simulink library "IsourcePower_lib"  (Simulink 8.1)
settings: Solver=ode45  SolverMode=SingleTasking  StartTime=0.0  StopTime=10.0  RelTol=1e-3
values from neighbouring files (symbols this model uses):
  Igrid = Pgrid/Vgrid/3    [Software_BESS_init.m]
  Ls_ess = Ls_ess_PU*Ls_ess_base    (= 0.000249351232441)    [Software_BESS_init.m]
  PUIMax = 1.2    [Software_BESS_init.m]
  Rs_ess = Rs_ess_PU*Rs_ess_base    (= 0.00497664)    [Software_BESS_init.m]
  sampdT = Tc    (= 0.0001)    [Software_BESS_init.m]
  Tc = Ts    (= 0.0001)    [Software_BESS_init.m]
  Ts = 100e-6    (= 0.0001)    [Software_BESS_init.m]
  Vgrid = 480/sqrt(3)    [Software_BESS_init.m]
undefined symbols (not defined in the file or in its folder): DiscIntNeverNeededParam, gcbh, sps, sps_rtmsupport
undefined symbols (not defined in the file): paramPLLControlD, paramPLLControlI, paramPLLControlP, PLLFreqChangeRateMax, PLLFreqCutOff
libraries: simulink x13, powerlib x12, powerlib_meascontrol x11, debounce_lib x8, powerlib_extras x7
settings Model: Creator=ch24070  LastModifiedBy=pkoralew  CovMetricSettings=dwe  CovHtmlReporting=off  covSaveCumulativeToWorkspaceVar=off  CovSaveSingleToWorkspaceVar=off  CovExternalEMLEnable=on

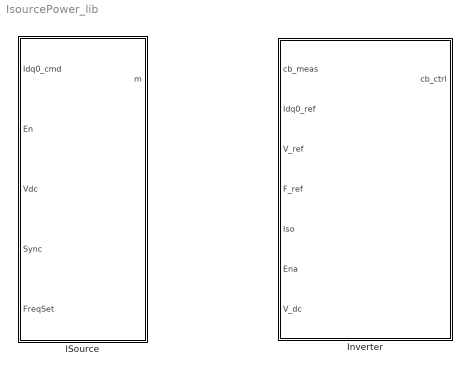
== system IsourcePower_lib ==
  ISource : Subsystem
  Inverter : Subsystem

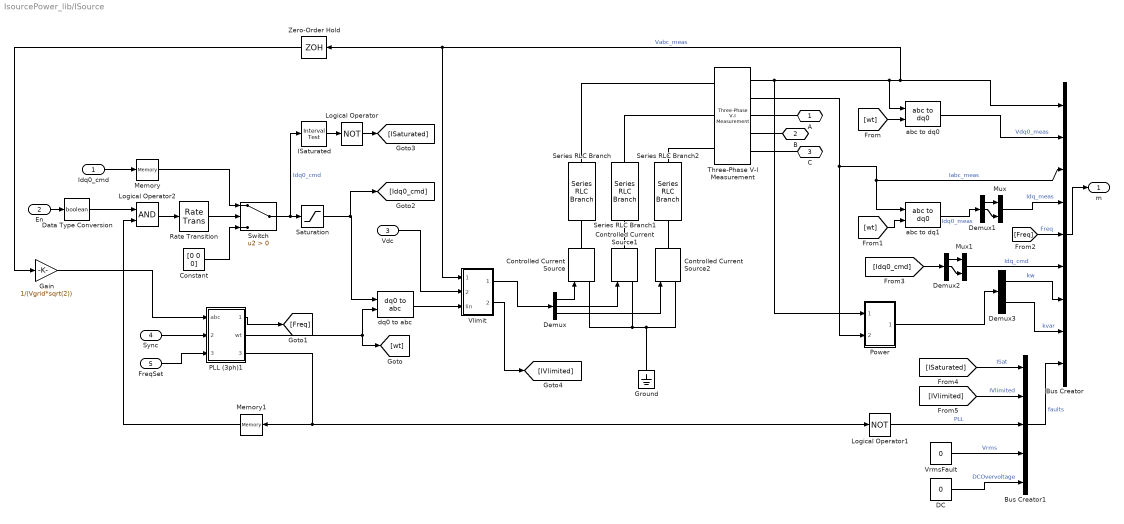
== system IsourcePower_lib/ISource ==
  Idq0_cmd : Inport
  En : Inport  Port=2
  Vdc : Inport  Port=3
  Sync : Inport  Port=4
  FreqSet : Inport  Port=5
  Bus Creator : BusCreator  Inputs=9
  Bus Creator1 : BusCreator  Inputs=5
  Constant : Constant  Value=[0 0 0]
  Controlled Current Source : powerlib/Electrical Sources/Controlled Current Source  Initialize=on  Source_Type=AC  Amplitude=0  Phase=0  Frequency=0  Measurements=None
  Controlled Current Source1 : powerlib/Electrical Sources/Controlled Current Source  Initialize=on  Source_Type=AC  Amplitude=0  Phase=0  Frequency=0  Measurements=None
  Controlled Current Source2 : powerlib/Electrical Sources/Controlled Current Source  Initialize=on  Source_Type=AC  Amplitude=0  Phase=0  Frequency=0  Measurements=None
  DC : Constant  Value=0
  Data Type Conversion : DataTypeConversion  OutDataTypeStr=boolean
  Demux : Demux  Outputs=3
  Demux1 : Demux  Outputs=3
  Demux2 : Demux  Outputs=3
  Demux3 : Demux  Outputs=2
  Gain : Gain  Gain=1/(Vgrid*sqrt(2))
  Ground : powerlib/Elements/Ground  LConnTagsString=a
  ISaturated : simulink/Logic and Bit Operations/Interval Test  IntervalClosedRight=on  uplimit=Igrid*sqrt(2)*PUIMax  IntervalClosedLeft=on  lowlimit=-Igrid*sqrt(2)*PUIMax  OutDataTypeStr=boolean
  Logical Operator : Logic  Operator=NOT  AllPortsSameDT=off  OutDataTypeStr=boolean
  Logical Operator1 : Logic  Operator=NOT  AllPortsSameDT=off  OutDataTypeStr=boolean
  Logical Operator2 : Logic  AllPortsSameDT=off  OutDataTypeStr=boolean
  Memory : Memory
  Memory1 : Memory
  Mux : Mux  Inputs=2
  Mux1 : Mux  Inputs=2
  PLL (3ph)1 : Subsystem  DialogController=POWERSYS.PowerSysDialog  LoadFcn=sps_rtmsupport('LoadFcn', gcbh);  StartFcn=sps_rtmsupport('StartFcn', gcbh);  StopFcn=sps_rtmsupport('StopFcn', gcbh);  mask(PLL (3ph)){Fmin=45, Par_Init=[0, 60], ParK=[paramPLLControlP, paramPLLControlI, paramPLLControlD], TcD=Tc, MaxRateChangeFreq=PLLFreqChangeRateMax, FilterCutOffFreq=PLLFreqCutOff, Ts=Tc, AGC=off}
      mask prompts: Fmin "Minimum frequency (Hz):"; Par_Init "Initial inputs [ Phase (degrees), Frequency (Hz) ]:"; ParK "Regulator gains [ Kp, Ki, Kd ]:"; TcD "Time constant for derivative action (s):"; MaxRateChangeFreq "Maximum rate of change of frequency (Hz/s):"; FilterCutOffFreq "Filter cut-off frequency for frequency measurement (Hz):"; Ts "Sample time:"; AGC "Enable automatic gain control"
      mask help:
      | This Phase Locked Loop (PLL) system can be used  to synchronize on a set of variable frequency, three-phase sinusoidal signals. If the Automatic Gain Control is enabled, the input (phase error) of the PLL regulator is scaled according to the input signals magnitude.
      |
      | For optimal performance, set regulator gains [ Kp Ki  Kd ] = [ 180  3200  1 ] and check the Enable Automatic Gain Control parameter.
      |
      | Input : Vector containing the normalized three-phase signals [Va Vb Vc]
      | Output 1:  Measured frequency (Hz) = w/(2pi)
      | Output 2:  Ramp w.t varying between  0 and 2*pi, synchronized on zero crossings of the fundamental (positive-sequence) of phase A.
      mask init:
      | %block=gcb;
      | %[WantBlockChoice,Ts,sps] = powericon('PLL3phInit',block,Fmin,Par_Init,ParK,TcD, MaxRateChangeFreq, FilterCutOffFreq, AGC,Ts);
      | %powericon('SetInternalModels','set',block,WantBlockChoice);
      settings: CopyFcn=sps_rtmsupport('CopyFcn', gcbh);  DeleteFcn=sps_rtmsupport('DeleteFcn', gcbh);  UndoDeleteFcn=sps_rtmsupport('UndoDeleteFcn', gcbh);  ModelCloseFcn=sps_rtmsupport('ModelCloseFcn', gcbh);  PreSaveFcn=sps_rtmsupport('PreSaveFcn', gcbh);  PostSaveFcn=sps_rtmsupport('PostSaveFcn', gcbh);  NameChangeFcn=sps_rtmsupport('NameChangeFcn', gcbh);  PreCopyFcn=sps_rtmsupport('PreCopyFcn', gcbh);  CloseFcn=sps_rtmsupport('CloseFcn', gcbh);  PreDeleteFcn=sps_rtmsupport('PreDeleteFcn', gcbh);
      settings: OpenFcn=|
      | power_openblockproxy();
      | sps_rtmsupport('OpenFcn', gcbh, [8]);
      mask Help: helpview(psbhelp);
  Power : Subsystem
  Rate Transition : RateTransition  OutPortSampleTime=Tc
  Saturation : Saturate  UpperLimit=Igrid*sqrt(2)*PUIMax  LowerLimit=-Igrid*sqrt(2)*PUIMax
  Series RLC Branch : powerlib/Elements/Series RLC Branch  LConnTagsString=__new0  RConnTagsString=__new0  BranchType=R  Resistance=1e-3  Inductance=0  SetiL0=off  InitialCurrent=0  Capacitance=0  Setx0=off  InitialVoltage=0  Measurements=None
  Series RLC Branch1 : powerlib/Elements/Series RLC Branch  LConnTagsString=__new0  RConnTagsString=__new0  BranchType=R  Resistance=1e-3  Inductance=0  SetiL0=off  InitialCurrent=0  Capacitance=0  Setx0=off  InitialVoltage=0  Measurements=None
  Series RLC Branch2 : powerlib/Elements/Series RLC Branch  LConnTagsString=__new0  RConnTagsString=__new0  BranchType=R  Resistance=1e-3  Inductance=0  SetiL0=off  InitialCurrent=0  Capacitance=0  Setx0=off  InitialVoltage=0  Measurements=None
  Switch : Switch  Criteria=u2 > Threshold
  Three-Phase V-I Measurement : powerlib/Measurements/Three-Phase V-I Measurement  VoltageMeasurement=phase-to-ground  SetLabelV=off  LabelV=Vabc  Vpu=off  VpuLL=off  CurrentMeasurement=yes  SetLabelI=off  LabelI=Iabc  Ipu=off  Pbase=100e6  Vbase=500e3  OutputType=Complex  PhasorSimulation=off  PSBequivalent=0
  Vlimit : Subsystem
  VrmsFault : Constant  Value=0
  Zero-Order Hold : ZeroOrderHold  SampleTime=Tc
  abc to dq0 : powerlib_meascontrol/Transformations/abc to dq0  Alignment=90 degrees behind phase A axis
  abc to dq1 : powerlib_meascontrol/Transformations/abc to dq0  Alignment=90 degrees behind phase A axis
  dq0 to abc : powerlib_meascontrol/Transformations/dq0 to abc  Alignment=90 degrees behind phase A axis
  A : PMIOPort  Port=1  Side=Right
  B : PMIOPort  Port=2  Side=Right
  C : PMIOPort  Port=3  Side=Right
  m : Outport
  wires:
  Memory1/1 -> Logical Operator2/2
  Data Type Conversion/1 -> Logical Operator2/1
  Logical Operator2/1 -> Rate Transition/1
  PLL (3ph)1/3(Lock) -> Logical Operator1/1, Memory1/1
  FreqSet/1 -> PLL (3ph)1/3(FreqSet)
  Sync/1 -> PLL (3ph)1/2(Sync)
  Logical Operator/1 -> [ISaturated]
  DC/1 -> Bus Creator1/5  "DCOvervoltage"
  Logical Operator1/1 -> Bus Creator1/3  "PLL"
  VrmsFault/1 -> Bus Creator1/4  "Vrms"
  [IVlimited] -> Bus Creator1/2  "IVlimited"
  Vlimit/2(Sat) -> [IVlimited]
  [ISaturated] -> Bus Creator1/1  "ISat"
  ISaturated/1 -> Logical Operator/1
  [Idq0_cmd] -> Demux2/1
  Power/1(Out1) -> Demux3/1
  Bus Creator1/1 -> Bus Creator/9  "faults"
  Vlimit/1(Ilim) -> Demux/1
  dq0 to abc/1 -> Vlimit/3(Iin)
  Vdc/1 -> Vlimit/2(Vdc)
  Saturation/1 -> dq0 to abc/1, [Idq0_cmd]
  Demux3/1 -> Bus Creator/7  "kw"
  Demux3/2 -> Bus Creator/8  "kvar"
  Bus Creator/1 -> m/1
  [Freq] -> Bus Creator/5  "Freq"
  Memory/1 -> Switch/1
  PLL (3ph)1/2(wt) -> dq0 to abc/2, [wt]
  Gain/1 -> PLL (3ph)1/1(abc)
  PLL (3ph)1/1(Freq) -> [Freq]
  Zero-Order Hold/1 -> Gain/1
  Constant/1 -> Switch/3
  En/1 -> Data Type Conversion/1
  abc to dq1/1 -> Demux1/1  "Idq0_meas"
  [wt] -> abc to dq1/2
  abc to dq0/1 -> Bus Creator/2  "Vdq0_meas"
  [wt] -> abc to dq0/2
  Three-Phase V-I Measurement/2 -> abc to dq1/1, Bus Creator/3, Power/2(In2)  "Iabc_meas"
  Three-Phase V-I Measurement/1 -> Zero-Order Hold/1, Vlimit/1(Vabc), Bus Creator/1, abc to dq0/1, Power/1(In1)  "Vabc_meas"
  Switch/1 -> Saturation/1, ISaturated/1  "Idq0_cmd"
  Demux/1 -> Controlled Current Source/1
  Demux/2 -> Controlled Current Source1/1
  Demux/3 -> Controlled Current Source2/1
  Rate Transition/1 -> Switch/2
  Demux1/1 -> Mux/1
  Demux1/2 -> Mux/2
  Demux2/1 -> Mux1/1
  Demux2/2 -> Mux1/2
  Mux1/1 -> Bus Creator/6  "Idq_cmd"
  Mux/1 -> Bus Creator/4  "Idq_meas"
  Idq0_cmd/1 -> Memory/1
  connections:
  Three-Phase V-I Measurement/RConn3 -- C/RConn1
  Three-Phase V-I Measurement/RConn1 -- A/RConn1
  Three-Phase V-I Measurement/RConn2 -- B/RConn1
  Three-Phase V-I Measurement/LConn1 -- Series RLC Branch/LConn1
  Three-Phase V-I Measurement/LConn3 -- Series RLC Branch2/LConn1
  Three-Phase V-I Measurement/LConn2 -- Series RLC Branch1/LConn1
  Controlled Current Source/RConn1 -- Series RLC Branch/RConn1
  Controlled Current Source1/RConn1 -- Series RLC Branch1/RConn1
  Controlled Current Source2/RConn1 -- Series RLC Branch2/RConn1
  Controlled Current Source/LConn1 -- Controlled Current Source1/LConn1 -- Controlled Current Source2/LConn1 -- Ground/LConn1

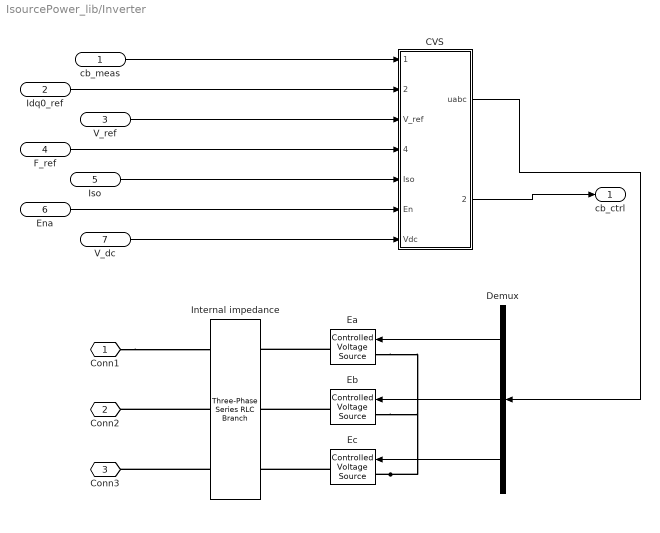
== system IsourcePower_lib/Inverter ==
  cb_meas : Inport
  Idq0_ref : Inport  Port=2
  V_ref : Inport  Port=3
  F_ref : Inport  Port=4
  Iso : Inport  Port=5
  Ena : Inport  Port=6
  V_dc : Inport  Port=7
  CVS : Subsystem
  Demux : Demux  Outputs=3
  Ea : powerlib/Electrical Sources/Controlled Voltage Source  Initialize=on  Source_Type=DC  Amplitude=0  Phase=0  Frequency=0  Measurements=None
  Eb : powerlib/Electrical Sources/Controlled Voltage Source  Initialize=on  Source_Type=DC  Amplitude=0  Phase=0  Frequency=0  Measurements=None
  Ec : powerlib/Electrical Sources/Controlled Voltage Source  Initialize=on  Source_Type=DC  Amplitude=0  Phase=0  Frequency=0  Measurements=None
  Internal impedance : powerlib/Elements/Three-Phase Series RLC Branch  LConnTagsString=A|B|C  RConnTagsString=A|B|C  BranchType=RL  Resistance=Rs_ess  Inductance=Ls_ess  Capacitance=1e-6  Measurements=None
  Conn1 : PMIOPort  Port=1  Side=Right
  Conn2 : PMIOPort  Port=2  Side=Right
  Conn3 : PMIOPort  Port=3  Side=Right
  cb_ctrl : Outport
  wires:
  V_ref/1 -> CVS/3(V_ref)
  cb_meas/1 -> CVS/1(cb_meas)
  CVS/2(cb_control) -> cb_ctrl/1
  Iso/1 -> CVS/5(Iso)
  V_dc/1 -> CVS/7(Vdc)
  F_ref/1 -> CVS/4(FreqSet)
  Ena/1 -> CVS/6(En)
  CVS/1(uabc) -> Demux/1
  Demux/1 -> Ea/1
  Demux/2 -> Eb/1
  Demux/3 -> Ec/1
  Idq0_ref/1 -> CVS/2(idq0_ref)
  connections:
  Ec/LConn1 -- Eb/LConn1 -- Ea/LConn1
  Ec/RConn1 -- Internal impedance/LConn3
  Eb/RConn1 -- Internal impedance/LConn2
  Ea/RConn1 -- Internal impedance/LConn1
  Conn1/RConn1 -- Internal impedance/RConn1
  Internal impedance/RConn2 -- Conn2/RConn1
  Internal impedance/RConn3 -- Conn3/RConn1

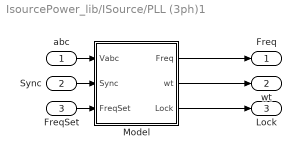
== system IsourcePower_lib/ISource/PLL (3ph)1 ==
  abc : Inport  PortDimensions=3  SampleTime=Ts
  Sync : Inport  Port=2  SampleTime=Ts
  FreqSet : Inport  Port=3  SampleTime=Ts
  Model : Subsystem  DialogController=POWERSYS.PowerSysDialog
  Freq : Outport  SampleTime=Ts
  wt : Outport  Port=2  SampleTime=Ts
  Lock : Outport  Port=3  SampleTime=Ts
  wires:
  Model/2(wt) -> wt/1
  Model/1(Freq) -> Freq/1
  FreqSet/1 -> Model/3(FreqSet)
  Sync/1 -> Model/2(Sync)
  abc/1 -> Model/1(Vabc)
  Model/3(Lock) -> Lock/1

== system IsourcePower_lib/ISource/Power ==
  In1 : Inport
  In2 : Inport  Port=2
  3-phase  Instantaneous  Active & Reactive Power : powerlib_extras/Measurements/3-phase  Instantaneous  Active & Reactive Power
  Discrete  Mean value2 : powerlib_extras/Discrete Measurements/Discrete  Mean value  Freq=60  Vinit=0  Ts=Ts
  Gain1 : Gain  Gain=(1/1000)
  Out1 : Outport
  wires:
  In1/1 -> 3-phase  Instantaneous  Active & Reactive Power/1
  In2/1 -> 3-phase  Instantaneous  Active & Reactive Power/2
  Gain1/1 -> Out1/1
  3-phase  Instantaneous  Active & Reactive Power/1 -> Discrete  Mean value2/1
  Discrete  Mean value2/1 -> Gain1/1

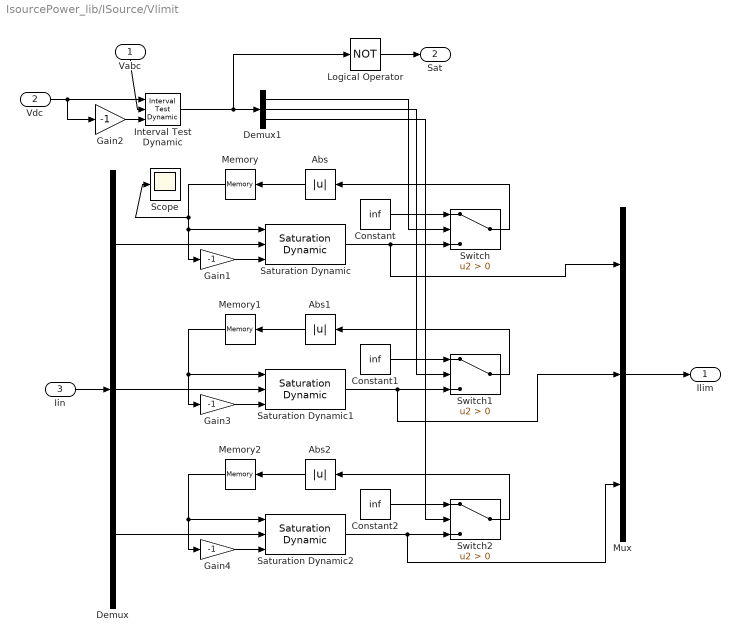
== system IsourcePower_lib/ISource/Vlimit ==
  Vabc : Inport
  Vdc : Inport  Port=2
  Iin : Inport  Port=3
  Abs : Abs
  Abs1 : Abs
  Abs2 : Abs
  Constant : Constant  Value=inf
  Constant1 : Constant  Value=inf
  Constant2 : Constant  Value=inf
  Demux : Demux  Outputs=3
  Demux1 : Demux  Outputs=3
  Gain{1..4} (4 alike) : Gain  Gain=-1
  Interval Test Dynamic : simulink/Logic and Bit Operations/Interval Test Dynamic  IntervalClosedRight=on  IntervalClosedLeft=on  OutDataTypeStr=boolean
  Logical Operator : Logic  Operator=NOT  AllPortsSameDT=off  OutDataTypeStr=boolean
  Memory : Memory
  Memory1 : Memory
  Memory2 : Memory
  Mux : Mux  Inputs=3
  Saturation Dynamic : simulink/Discontinuities/Saturation Dynamic  OutMin=[]  OutMax=[]  OutDataTypeStr=Inherit: Same as second input  OutDataType=fixdt(1, 16)  OutScaling=2^-10  RndMeth=Round  DoSatur=off
  Saturation Dynamic1 : simulink/Discontinuities/Saturation Dynamic  OutMin=[]  OutMax=[]  OutDataTypeStr=Inherit: Same as second input  OutDataType=fixdt(1, 16)  OutScaling=2^-10  DoSatur=off
  Saturation Dynamic2 : simulink/Discontinuities/Saturation Dynamic  OutMin=[]  OutMax=[]  OutDataTypeStr=Inherit: Same as second input  OutDataType=fixdt(1, 16)  OutScaling=2^-10  DoSatur=off
  Scope : Scope
      settings: YMin=-22.88103  YMax=205.92926
  Switch : Switch  Criteria=u2 > Threshold
  Switch1 : Switch  Criteria=u2 > Threshold
  Switch2 : Switch  Criteria=u2 > Threshold
  Ilim : Outport
  Sat : Outport  Port=2
  wires:
  Logical Operator/1 -> Sat/1
  Vabc/1 -> Interval Test Dynamic/2
  Vdc/1 -> Gain2/1, Interval Test Dynamic/1
  Gain2/1 -> Interval Test Dynamic/3
  Mux/1 -> Ilim/1
  Abs/1 -> Memory/1
  Gain1/1 -> Saturation Dynamic/3
  Saturation Dynamic/1 -> Mux/1, Switch/3
  Constant/1 -> Switch/1
  Switch/1 -> Abs/1
  Iin/1 -> Demux/1
  Demux1/1 -> Switch/2
  Demux/1 -> Saturation Dynamic/2
  Abs1/1 -> Memory1/1
  Gain3/1 -> Saturation Dynamic1/3
  Saturation Dynamic1/1 -> Mux/2, Switch1/3
  Constant1/1 -> Switch1/1
  Switch1/1 -> Abs1/1
  Demux/2 -> Saturation Dynamic1/2
  Abs2/1 -> Memory2/1
  Gain4/1 -> Saturation Dynamic2/3
  Saturation Dynamic2/1 -> Mux/3, Switch2/3
  Constant2/1 -> Switch2/1
  Demux/3 -> Saturation Dynamic2/2
  Demux1/2 -> Switch1/2
  Demux1/3 -> Switch2/2
  Switch2/1 -> Abs2/1
  Memory/1 -> Scope/1, Gain1/1, Saturation Dynamic/1
  Memory1/1 -> Gain3/1, Saturation Dynamic1/1
  Memory2/1 -> Saturation Dynamic2/1, Gain4/1
  Interval Test Dynamic/1 -> Demux1/1, Logical Operator/1

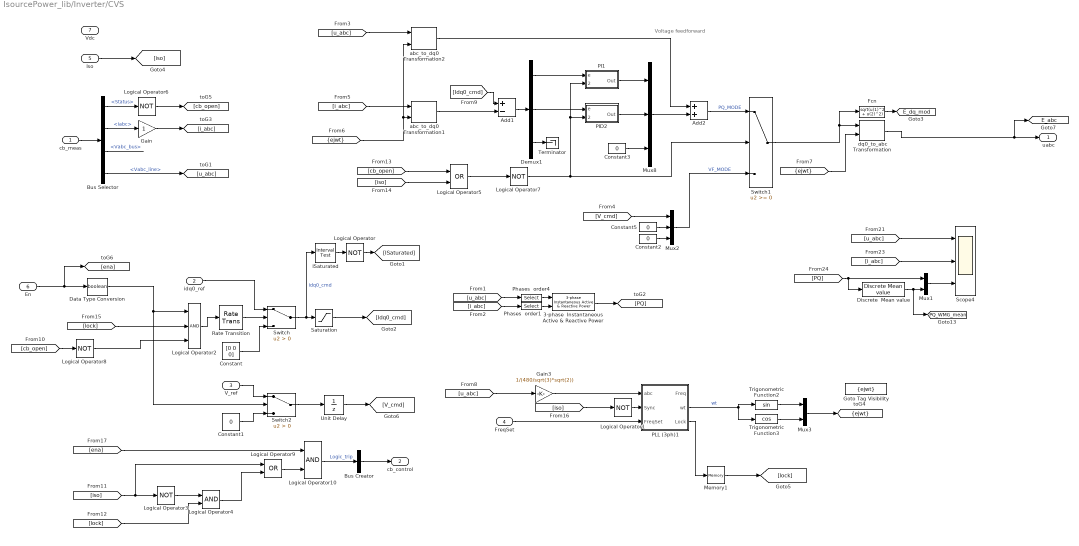
== system IsourcePower_lib/Inverter/CVS ==
  note: Voltage feedforward
  cb_meas : Inport
  idq0_ref : Inport  Port=2
  V_ref : Inport  Port=3
  FreqSet : Inport  Port=4
  Iso : Inport  Port=5
  En : Inport  Port=6
  Vdc : Inport  Port=7
  3-phase  Instantaneous  Active & Reactive Power : powerlib_extras/Measurements/3-phase  Instantaneous  Active & Reactive Power
  Add1 : Sum  Inputs=+-
  Add2 : Sum
  Bus Creator : BusCreator  Inputs=1
  Bus Selector : BusSelector  OutputSignals=Status,Iabc,Vabc_bus,Vabc_line
  Constant : Constant  Value=[0 0 0]
  Constant{1..3,5} (4 alike) : Constant  Value=0
  Data Type Conversion : DataTypeConversion  OutDataTypeStr=boolean
  Demux1 : Demux  Outputs=3
  Discrete  Mean value : powerlib_extras/Discrete Measurements/Discrete  Mean value  Freq=60*10  Vinit=0  Ts=Ts
  Fcn : Fcn  Expr=sqrt(u(1)^2 + u(2)^2)
  Gain : Gain
  Gain3 : Gain  Gain=1/(480/sqrt(3)*sqrt(2))
  Goto Tag Visibility : GotoTagVisibility  GotoTag=ejwt
  ISaturated : simulink/Logic and Bit Operations/Interval Test  IntervalClosedRight=on  uplimit=Igrid*sqrt(2)*PUIMax  IntervalClosedLeft=on  lowlimit=-Igrid*sqrt(2)*PUIMax  OutDataTypeStr=boolean
  Logical Operator{,1,3,6..8} (6 alike) : Logic  Operator=NOT  AllPortsSameDT=off  OutDataTypeStr=boolean
  Logical Operator10 : Logic  AllPortsSameDT=off  OutDataTypeStr=boolean
  Logical Operator2 : Logic  Inputs=3  AllPortsSameDT=off  OutDataTypeStr=boolean
  Logical Operator4 : Logic  AllPortsSameDT=off  OutDataTypeStr=boolean
  Logical Operator5 : Logic  Operator=OR  AllPortsSameDT=off  OutDataTypeStr=boolean
  Logical Operator9 : Logic  Operator=OR  AllPortsSameDT=off  OutDataTypeStr=boolean
  Memory1 : Memory
  Mux1 : Mux  Inputs=2
  Mux2 : Mux  Inputs=3
  Mux3 : Mux  Inputs=2
  Mux8 : Mux  Inputs=3
  PI1 : Subsystem  mask{Kp=0.4*5, Ti=3e-3/5, Ts=Ts, D=0, Iup=1e3, Idown=-1e3, PIup=1e3, PIdown=-1e3, Int_init=0, Enable_zero_val=0}
      mask prompts: Kp "Proportional gain Kp"; Ti "Integral doubling-time Ti [s]"; Ts "Sample time [s]"; D "Derivative Gain"; Iup "Integral upper saturation limit"; Idown "Integral lower saturation limit"; PIup "PI output upper saturation limit"; PIdown "PI output lower saturation limit"; Int_init "Integral initial value"; Enable_zero_val "Output value when Enable=0"
      mask help: PID controller integral is in enable state when Enable signal value equals 1. If Enable state equals zero the PID output also equals zero.
  PID2 : Subsystem  mask{Kp=0.4*5, Ti=3e-3/5, Ts=Ts, D=0, Iup=1e3, Idown=-1e3, PIup=1e3, PIdown=-1e3, Int_init=0, Enable_zero_val=0}
      mask prompts: Kp "Proportional gain Kp"; Ti "Integral doubling-time Ti [s]"; Ts "Sample time [s]"; D "Derivative Gain"; Iup "Integral upper saturation limit"; Idown "Integral lower saturation limit"; PIup "PI output upper saturation limit"; PIdown "PI output lower saturation limit"; Int_init "Integral initial value"; Enable_zero_val "Output value when Enable=0"
      mask help: PID controller integral is in enable state when Enable signal value equals 1. If Enable state equals zero the PID output also equals zero.
  PLL (3ph)1 : Subsystem  DialogController=POWERSYS.PowerSysDialog  LoadFcn=sps_rtmsupport('LoadFcn', gcbh);  StartFcn=sps_rtmsupport('StartFcn', gcbh);  StopFcn=sps_rtmsupport('StopFcn', gcbh);  mask(PLL (3ph)){Fmin=45, Par_Init=[0, 60], ParK=[paramPLLControlP, paramPLLControlI, paramPLLControlD], TcD=Tc, MaxRateChangeFreq=PLLFreqChangeRateMax, FilterCutOffFreq=PLLFreqCutOff, Ts=Ts, AGC=off}
      mask prompts: Fmin "Minimum frequency (Hz):"; Par_Init "Initial inputs [ Phase (degrees), Frequency (Hz) ]:"; ParK "Regulator gains [ Kp, Ki, Kd ]:"; TcD "Time constant for derivative action (s):"; MaxRateChangeFreq "Maximum rate of change of frequency (Hz/s):"; FilterCutOffFreq "Filter cut-off frequency for frequency measurement (Hz):"; Ts "Sample time:"; AGC "Enable automatic gain control"
      mask help:
      | This Phase Locked Loop (PLL) system can be used  to synchronize on a set of variable frequency, three-phase sinusoidal signals. If the Automatic Gain Control is enabled, the input (phase error) of the PLL regulator is scaled according to the input signals magnitude.
      |
      | For optimal performance, set regulator gains [ Kp Ki  Kd ] = [ 180  3200  1 ] and check the Enable Automatic Gain Control parameter.
      |
      | Input : Vector containing the normalized three-phase signals [Va Vb Vc]
      | Output 1:  Measured frequency (Hz) = w/(2pi)
      | Output 2:  Ramp w.t varying between  0 and 2*pi, synchronized on zero crossings of the fundamental (positive-sequence) of phase A.
      mask init:
      | %block=gcb;
      | %[WantBlockChoice,Ts,sps] = powericon('PLL3phInit',block,Fmin,Par_Init,ParK,TcD, MaxRateChangeFreq, FilterCutOffFreq, AGC,Ts);
      | %powericon('SetInternalModels','set',block,WantBlockChoice);
      settings: CopyFcn=sps_rtmsupport('CopyFcn', gcbh);  DeleteFcn=sps_rtmsupport('DeleteFcn', gcbh);  UndoDeleteFcn=sps_rtmsupport('UndoDeleteFcn', gcbh);  ModelCloseFcn=sps_rtmsupport('ModelCloseFcn', gcbh);  PreSaveFcn=sps_rtmsupport('PreSaveFcn', gcbh);  PostSaveFcn=sps_rtmsupport('PostSaveFcn', gcbh);  NameChangeFcn=sps_rtmsupport('NameChangeFcn', gcbh);  PreCopyFcn=sps_rtmsupport('PreCopyFcn', gcbh);  CloseFcn=sps_rtmsupport('CloseFcn', gcbh);  PreDeleteFcn=sps_rtmsupport('PreDeleteFcn', gcbh);
      settings: OpenFcn=|
      | power_openblockproxy();
      | sps_rtmsupport('OpenFcn', gcbh, [8]);
      mask Help: helpview(psbhelp);
  Phases  order1 : Selector  InputPortWidth=3  IndexOptions=Index vector (dialog)  Indices=[1 3 2]  OutputSizes=1
  Phases  order4 : Selector  InputPortWidth=3  IndexOptions=Index vector (dialog)  Indices=[1 3 2]  OutputSizes=1
  Rate Transition : RateTransition  OutPortSampleTime=Tc
  Saturation : Saturate  UpperLimit=Igrid*sqrt(2)*PUIMax  LowerLimit=-Igrid*sqrt(2)*PUIMax
  Scope4 : Scope  NumInputPorts=3
      settings: TimeRange=0.4  YMin=-400~-1500~-650000  YMax=400~1500~-325000  SaveName=ScopeData9  MaxDataPoints=100e3
  Switch : Switch  Criteria=u2 > Threshold
  Switch1 : Switch
  Switch2 : Switch  Criteria=u2 > Threshold
  Terminator : Terminator
  Trigonometric Function2 : Trigonometry
  Trigonometric Function3 : Trigonometry  Operator=cos
  Unit Delay : UnitDelay  SampleTime=-1
  abc_to_dq0 Transformation1 : powerlib_extras/Measurements/abc_to_dq0 Transformation
  abc_to_dq0 Transformation2 : powerlib_extras/Measurements/abc_to_dq0 Transformation
  dq0_to_abc Transformation : powerlib_extras/Measurements/dq0_to_abc Transformation
  uabc : Outport
  cb_control : Outport  Port=2
  tag scope: E_abc=global, E_dq_mod=global, PQ_WMG_mean=global, ejwt=scoped
  wires:
  Logical Operator10/1 -> Bus Creator/1  "Logic_trip"
  [ena] -> Logical Operator10/1
  Logical Operator9/1 -> Logical Operator10/2
  [i_abc] -> abc_to_dq0 Transformation1/1
  [u_abc] -> abc_to_dq0 Transformation2/1
  Unit Delay/1 -> [V_cmd]
  [iso] -> Logical Operator1/1
  Constant1/1 -> Switch2/3
  V_ref/1 -> Switch2/1
  Data Type Conversion/1 -> Logical Operator2/1, Switch2/2
  Switch2/1 -> Unit Delay/1
  Iso/1 -> [iso]
  Add2/1 -> Switch1/1  "PQ_MODE"
  Mux8/1 -> Add2/2
  abc_to_dq0 Transformation2/1 -> Add2/1
  [lock] -> Logical Operator2/2
  Memory1/1 -> [lock]
  Demux1/3 -> Terminator/1
  [Idq0_cmd] -> Add1/1
  Gain/1 -> [i_abc]
  Bus Selector/4 -> [u_abc]  "<Vabc_line>"
  Bus Selector/3 -> ?  "<Vabc_bus>"
  Saturation/1 -> [Idq0_cmd]
  Logical Operator8/1 -> Logical Operator2/3
  [cb_open] -> Logical Operator8/1
  [cb_open] -> Logical Operator5/1
  Logical Operator6/1 -> [cb_open]
  Bus Selector/1 -> Logical Operator6/1  "<Status>"
  [iso] -> Logical Operator5/2
  Logical Operator4/1 -> Logical Operator9/2
  Bus Creator/1 -> cb_control/1
  [lock] -> Logical Operator4/2
  Logical Operator3/1 -> Logical Operator4/1
  [iso] -> Logical Operator3/1, Logical Operator9/1
  Logical Operator1/1 -> PLL (3ph)1/2(Sync)
  Logical Operator7/1 -> PID2/2(Enable), PI1/2(Enable), Switch1/2
  Gain3/1 -> PLL (3ph)1/1(abc)
  Logical Operator2/1 -> Rate Transition/1
  Logical Operator/1 -> [ISaturated]
  ISaturated/1 -> Logical Operator/1
  Constant/1 -> Switch/3
  En/1 -> Data Type Conversion/1, [ena]
  Switch/1 -> Saturation/1, ISaturated/1  "Idq0_cmd"
  Rate Transition/1 -> Switch/2
  PLL (3ph)1/3(Lock) -> Memory1/1
  FreqSet/1 -> PLL (3ph)1/3(FreqSet)
  Trigonometric Function3/1 -> Mux3/2
  Trigonometric Function2/1 -> Mux3/1
  PLL (3ph)1/2(wt) -> Trigonometric Function3/1, Trigonometric Function2/1  "wt"
  [u_abc] -> Gain3/1
  Add1/1 -> Demux1/1
  Constant3/1 -> Mux8/3
  Constant2/1 -> Mux2/3
  Demux1/2 -> PID2/1(e)
  Demux1/1 -> PI1/1(e)
  Mux2/1 -> Switch1/3  "VF_MODE"
  Constant5/1 -> Mux2/2
  [V_cmd] -> Mux2/1
  Logical Operator5/1 -> Logical Operator7/1
  PID2/1(Out) -> Mux8/2
  PI1/1(Out) -> Mux8/1
  Switch1/1 -> dq0_to_abc Transformation/1, Fcn/1
  Fcn/1 -> [E_dq_mod]
  [ejwt] -> abc_to_dq0 Transformation1/2, abc_to_dq0 Transformation2/2
  [ejwt] -> dq0_to_abc Transformation/2
  idq0_ref/1 -> Switch/1
  abc_to_dq0 Transformation1/1 -> Add1/2
  Phases  order1/1 -> 3-phase  Instantaneous  Active & Reactive Power/2
  Phases  order4/1 -> 3-phase  Instantaneous  Active & Reactive Power/1
  Bus Selector/2 -> Gain/1  "<Iabc>"
  cb_meas/1 -> Bus Selector/1
  Mux1/1 -> Scope4/3
  Discrete  Mean value/1 -> [PQ_WMG_mean], Mux1/2
  [PQ] -> Mux1/1, Discrete  Mean value/1
  [i_abc] -> Scope4/2
  [u_abc] -> Scope4/1
  3-phase  Instantaneous  Active & Reactive Power/1 -> [PQ]
  [i_abc] -> Phases  order1/1
  [u_abc] -> Phases  order4/1
  dq0_to_abc Transformation/1 -> [E_abc], uabc/1
  Mux3/1 -> [ejwt]

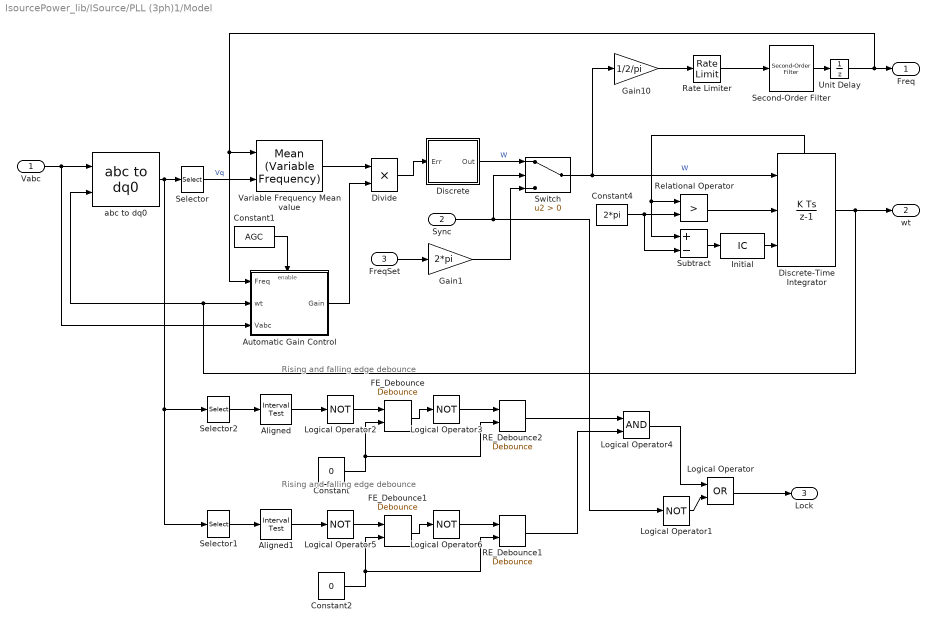
== system IsourcePower_lib/ISource/PLL (3ph)1/Model ==
  note: Rising and falling edge debounce
  note: Rising and falling edge debounce
  Vabc : Inport  PortDimensions=3
  Sync : Inport  Port=2
  FreqSet : Inport  Port=3
  Aligned : simulink/Logic and Bit Operations/Interval Test  IntervalClosedRight=on  uplimit=0.05  IntervalClosedLeft=on  lowlimit=-0.05  OutDataTypeStr=boolean
  Aligned1 : simulink/Logic and Bit Operations/Interval Test  IntervalClosedRight=on  uplimit=1.05  IntervalClosedLeft=on  lowlimit=-1.05  OutDataTypeStr=boolean
  Automatic Gain Control : Subsystem  TreatAsAtomicUnit=on
  Constant : Constant  Value=0
  Constant1 : Constant  Value=AGC  SampleTime=Ts
  Constant2 : Constant  Value=0
  Constant4 : Constant  Value=2*pi  SampleTime=Ts
  Discrete : Subsystem  DialogController=POWERSYS.PowerSysDialog  VariantControl=PID_Discrete  mask(Discrete PID Controller){Kp=ParK(1), Ki=ParK(2), Kd=ParK(3), TcD=TcD, Par_Limits=[inf 0], Init=2*pi*Par_Init(2), Ts=Ts}
      mask prompts: Kp "Proportional gain (Kp):"; Ki "Integral gain (Ki):"; Kd "Derivative gain (Kd):"; TcD "Time constant for derivative filter (s):"; Par_Limits "Output limits: [ Upper   Lower ]"; Init "Output initial value:"; Ts "Sample time:"
      mask help: This block implements a discrete PID controller.
      mask Display: disp('PID');
  Discrete-Time Integrator : DiscreteIntegrator  ExternalReset=rising  InitialConditionSource=external  InitialCondition=sps.Phase_Init*pi/180  InitialConditionMode=State only (most efficient)  SampleTime=Ts  ShowStatePort=on  ICPrevOutput=DiscIntNeverNeededParam  ICPrevScaledInput=DiscIntNeverNeededParam
  Divide : Product
  FE_Debounce : debounce_lib/Debounce  Ts=sampdT  Td=paramPLLQFEDebounceTime
  FE_Debounce1 : debounce_lib/Debounce  Ts=sampdT  Td=paramPLLQFEDebounceTime
  Gain1 : Gain  Gain=2*pi  SaturateOnIntegerOverflow=on  OutDataTypeStr=Inherit: Same as input  ParamDataTypeStr=Inherit: Same as input
  Gain10 : Gain  Gain=1/2/pi  SaturateOnIntegerOverflow=on  OutDataTypeStr=Inherit: Same as input  ParamDataTypeStr=Inherit: Same as input
  Initial : InitialCondition  Value=0
  Logical Operator : Logic  Operator=OR  AllPortsSameDT=off  OutDataTypeStr=boolean
  Logical Operator1 : Logic  Operator=NOT  AllPortsSameDT=off  OutDataTypeStr=boolean
  Logical Operator{2..3,5..6} (4 alike) : Logic  Operator=NOT  Inputs=1  AllPortsSameDT=off  OutDataTypeStr=boolean
  Logical Operator4 : Logic  AllPortsSameDT=off  OutDataTypeStr=boolean
  RE_Debounce1 : debounce_lib/Debounce  Ts=sampdT  Td=1
  RE_Debounce2 : debounce_lib/Debounce  Ts=sampdT  Td=1
  Rate Limiter : RateLimiter  RisingSlewLimit=MaxRateChangeFreq  FallingSlewLimit=-MaxRateChangeFreq  SampleTimeMode=inherited  InitialCondition=Par_Init(2)
  Relational Operator : RelationalOperator  Operator=>  OutDataTypeStr=boolean
  Second-Order Filter : powerlib_meascontrol/Filters/Second-Order Filter  FilterType=Lowpass  Fo=FilterCutOffFreq  Zeta=0.707  Ts=Ts  Initialize=on  Vac_Init=[0 0 Par_Init(2)]  Vdc_Init=Par_Init(2)  PlotResponse=off  FreqRange=[1 500 1]
  Selector : Selector  InputPortWidth=3  IndexOptions=Index vector (dialog)  Indices=2  OutputSizes=1
  Selector1 : Selector  InputPortWidth=3  IndexOptions=Index vector (dialog)  Indices=1  OutputSizes=1
  Selector2 : Selector  InputPortWidth=3  IndexOptions=Index vector (dialog)  Indices=2  OutputSizes=1
  Subtract : Sum  Inputs=+-
  Switch : Switch  Criteria=u2 > Threshold
  Unit Delay : UnitDelay  InitialCondition=Par_Init(2)  SampleTime=Ts
  Variable Frequency Mean value : powerlib_meascontrol/Measurements/Mean (Variable Frequency)  Finit=Par_Init(2)  Fmin=Fmin  Vinit=0  Ts=Ts
  abc to dq0 : powerlib_meascontrol/Transformations/abc to dq0  Alignment=90 degrees behind phase A axis
  Freq : Outport
  wt : Outport  Port=2
  Lock : Outport  Port=3
  wires:
  Logical Operator4/1 -> Logical Operator/1
  RE_Debounce1/1 -> Logical Operator4/2
  Selector1/1 -> Aligned1/1
  Aligned1/1 -> Logical Operator5/1
  Constant2/1 -> RE_Debounce1/2, FE_Debounce1/2
  Logical Operator6/1 -> RE_Debounce1/1
  FE_Debounce1/1 -> Logical Operator6/1
  Logical Operator5/1 -> FE_Debounce1/1
  RE_Debounce2/1 -> Logical Operator4/1
  Selector2/1 -> Aligned/1
  Aligned/1 -> Logical Operator2/1
  Constant/1 -> FE_Debounce/2, RE_Debounce2/2
  Logical Operator3/1 -> RE_Debounce2/1
  FE_Debounce/1 -> Logical Operator3/1
  Logical Operator2/1 -> FE_Debounce/1
  Logical Operator1/1 -> Logical Operator/2
  Logical Operator/1 -> Lock/1
  Gain1/1 -> Switch/3
  Discrete/1(Out) -> Switch/1  "W"
  Sync/1 -> Switch/2, Logical Operator1/1
  FreqSet/1 -> Gain1/1
  Unit Delay/1 -> Freq/1, Automatic Gain Control/1(Freq), Variable Frequency Mean value/1
  Rate Limiter/1 -> Second-Order Filter/1
  Gain10/1 -> Rate Limiter/1
  Selector/1 -> Variable Frequency Mean value/2  "Vq"
  Second-Order Filter/1 -> Unit Delay/1
  Discrete-Time Integrator/1 -> abc to dq0/2, Automatic Gain Control/2(wt), wt/1
  Constant4/1 -> Subtract/2, Relational Operator/2
  abc to dq0/1 -> Selector/1, Selector1/1, Selector2/1
  Vabc/1 -> abc to dq0/1, Automatic Gain Control/3(Vabc)
  Switch/1 -> Gain10/1, Discrete-Time Integrator/1  "W"
  Variable Frequency Mean value/1 -> Divide/1
  Automatic Gain Control/1(Gain) -> Divide/2
  Divide/1 -> Discrete/1(Err)
  Constant1/1 -> Automatic Gain Control/Enable
  Relational Operator/1 -> Discrete-Time Integrator/2
  Discrete-Time Integrator/State -> Subtract/1, Relational Operator/1
  Subtract/1 -> Initial/1
  Initial/1 -> Discrete-Time Integrator/3

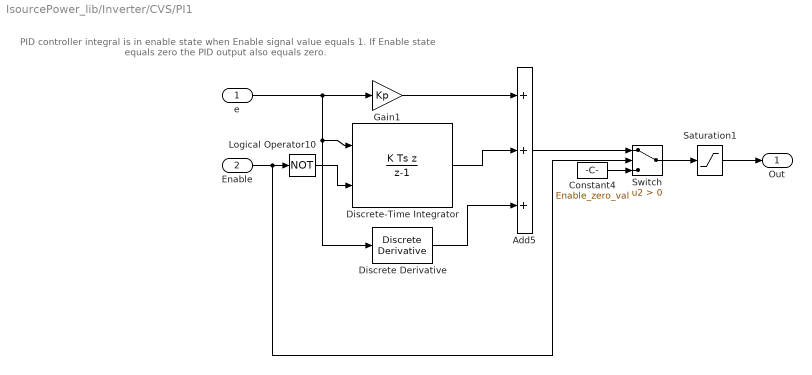
== system IsourcePower_lib/Inverter/CVS/PI1 ==
  note: PID controller integral is in enable state when Enable signal value equals 1. If Enable state equals zero the PID output also equals zero.
  e : Inport
  Enable : Inport  Port=2
  Add5 : Sum  Inputs=+++
  Constant4 : Constant  Value=Enable_zero_val
  Discrete Derivative : simulink/Discrete/Discrete Derivative  gainval=D  ICPrevScaledInput=0.0  InputProcessing=Inherited  OutMin=[]  OutMax=[]  OutDataType=fixdt(1, 16)  OutScaling=2^-10  DoSatur=off
  Discrete-Time Integrator : DiscreteIntegrator  IntegratorMethod=Integration: Backward Euler  gainval=1/Ti  ExternalReset=level  InitialCondition=Int_init  SampleTime=Ts  LimitOutput=on  UpperSaturationLimit=Iup  LowerSaturationLimit=Idown  ICPrevOutput=DiscIntNeverNeededParam  ICPrevScaledInput=DiscIntNeverNeededParam
  Gain1 : Gain  Gain=Kp
  Logical Operator10 : Logic  Operator=NOT  IconShape=distinctive  AllPortsSameDT=off  OutDataTypeStr=boolean
  Saturation1 : Saturate  UpperLimit=PIup  LowerLimit=PIdown  LinearizeAsGain=off
  Switch : Switch  Criteria=u2 > Threshold
  Out : Outport
  wires:
  ? -> ?
  Discrete Derivative/1 -> Add5/3
  Add5/1 -> Switch/1
  Constant4/1 -> Switch/3
  Logical Operator10/1 -> Discrete-Time Integrator/2
  e/1 -> Discrete Derivative/1, Discrete-Time Integrator/1, Gain1/1
  Discrete-Time Integrator/1 -> Add5/2
  Gain1/1 -> Add5/1
  Enable/1 -> Switch/2, Logical Operator10/1
  Switch/1 -> Saturation1/1
  Saturation1/1 -> Out/1

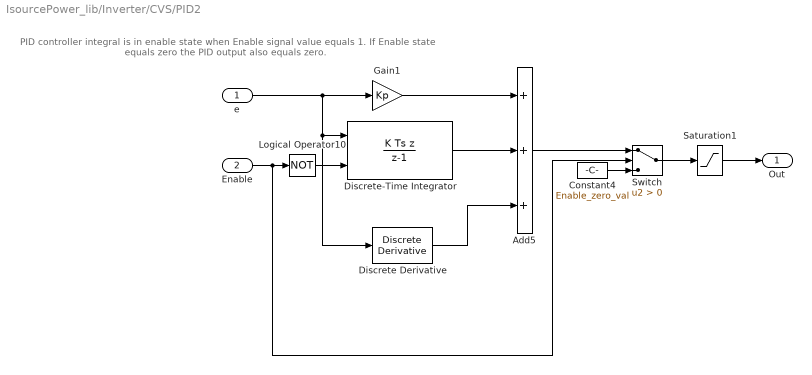
== system IsourcePower_lib/Inverter/CVS/PID2 ==
  note: PID controller integral is in enable state when Enable signal value equals 1. If Enable state equals zero the PID output also equals zero.
  e : Inport
  Enable : Inport  Port=2
  Add5 : Sum  Inputs=+++
  Constant4 : Constant  Value=Enable_zero_val
  Discrete Derivative : simulink/Discrete/Discrete Derivative  gainval=D  ICPrevScaledInput=0.0  InputProcessing=Inherited  OutMin=[]  OutMax=[]  OutDataType=fixdt(1, 16)  OutScaling=2^-10  DoSatur=off
  Discrete-Time Integrator : DiscreteIntegrator  IntegratorMethod=Integration: Backward Euler  gainval=1/Ti  ExternalReset=level  InitialCondition=Int_init  SampleTime=Ts  LimitOutput=on  UpperSaturationLimit=Iup  LowerSaturationLimit=Idown  ICPrevOutput=DiscIntNeverNeededParam  ICPrevScaledInput=DiscIntNeverNeededParam
  Gain1 : Gain  Gain=Kp
  Logical Operator10 : Logic  Operator=NOT  IconShape=distinctive  AllPortsSameDT=off  OutDataTypeStr=boolean
  Saturation1 : Saturate  UpperLimit=PIup  LowerLimit=PIdown  LinearizeAsGain=off
  Switch : Switch  Criteria=u2 > Threshold
  Out : Outport
  wires:
  Saturation1/1 -> Out/1
  Switch/1 -> Saturation1/1
  Enable/1 -> Logical Operator10/1, Switch/2
  Gain1/1 -> Add5/1
  Discrete-Time Integrator/1 -> Add5/2
  e/1 -> Gain1/1, Discrete-Time Integrator/1, Discrete Derivative/1
  Logical Operator10/1 -> Discrete-Time Integrator/2
  Constant4/1 -> Switch/3
  Add5/1 -> Switch/1
  Discrete Derivative/1 -> Add5/3

== system IsourcePower_lib/Inverter/CVS/PLL (3ph)1 ==
  abc : Inport  PortDimensions=3  SampleTime=Ts
  Sync : Inport  Port=2  SampleTime=Ts
  FreqSet : Inport  Port=3  SampleTime=Ts
  Model : Subsystem  DialogController=POWERSYS.PowerSysDialog
  Freq : Outport  SampleTime=Ts
  wt : Outport  Port=2  SampleTime=Ts
  Lock : Outport  Port=3  SampleTime=Ts
  wires:
  Model/2(wt) -> wt/1
  Model/1(Freq) -> Freq/1
  FreqSet/1 -> Model/3(FreqSet)
  Sync/1 -> Model/2(Sync)
  abc/1 -> Model/1(Vabc)
  Model/3(Lock) -> Lock/1

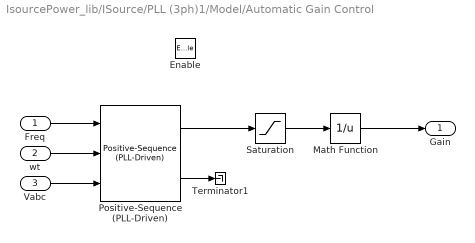
== system IsourcePower_lib/ISource/PLL (3ph)1/Model/Automatic Gain Control ==
  Freq : Inport
  wt : Inport  Port=2
  Vabc : Inport  Port=3
  Enable : EnablePort  PropagateVarSize=During execution
  Math Function : Math  Operator=reciprocal  SaturateOnIntegerOverflow=on
  Positive-Sequence (PLL-Driven) : powerlib_meascontrol/Measurements/Positive-Sequence (PLL-Driven)  Finit=Par_Init(2)  Fmin=Fmin  InInit=[1 0]  Ts=Ts
  Saturation : Saturate  UpperLimit=inf  LowerLimit=eps
  Terminator1 : Terminator
  Gain : Outport  InitialOutput=[1]
  wires:
  Positive-Sequence (PLL-Driven)/1 -> Saturation/1
  Positive-Sequence (PLL-Driven)/2 -> Terminator1/1
  wt/1 -> Positive-Sequence (PLL-Driven)/2
  Math Function/1 -> Gain/1
  Vabc/1 -> Positive-Sequence (PLL-Driven)/3
  Freq/1 -> Positive-Sequence (PLL-Driven)/1
  Saturation/1 -> Math Function/1

== system IsourcePower_lib/ISource/PLL (3ph)1/Model/Discrete ==
  Err : Inport  SampleTime=Ts
  "Discrete Derivative " : DiscreteTransferFcn  Numerator="[ 1  -1 ]*Kd"  Denominator="[ TcD  Ts-TcD ]"  SampleTime=Ts
  Discrete-Time Integrator : DiscreteIntegrator  gainval=Ki  InitialCondition=Init  SampleTime=Ts  LimitOutput=on  UpperSaturationLimit=Par_Limits(1)  LowerSaturationLimit=Par_Limits(2)  ICPrevOutput=DiscIntNeverNeededParam  ICPrevScaledInput=DiscIntNeverNeededParam
  Kp4 : Gain  Gain=Kp  SampleTime=Ts  SaturateOnIntegerOverflow=on  OutDataTypeStr=Inherit: Same as input  ParamDataTypeStr=Inherit: Same as input
  Saturation1 : Saturate  UpperLimit=Par_Limits(1)  LowerLimit=Par_Limits(2)  SampleTime=Ts
  Sum6 : Sum  Inputs=+++  SampleTime=Ts  SaturateOnIntegerOverflow=on  InputSameDT=on  OutDataTypeStr=Inherit: Same as first input
  Out : Outport  SampleTime=Ts  InitialOutput=0
  wires:
  "Discrete Derivative "/1 -> Sum6/3
  Discrete-Time Integrator/1 -> Sum6/2
  Kp4/1 -> Sum6/1
  Sum6/1 -> Saturation1/1
  Err/1 -> Kp4/1, Discrete-Time Integrator/1, "Discrete Derivative "/1
  Saturation1/1 -> Out/1

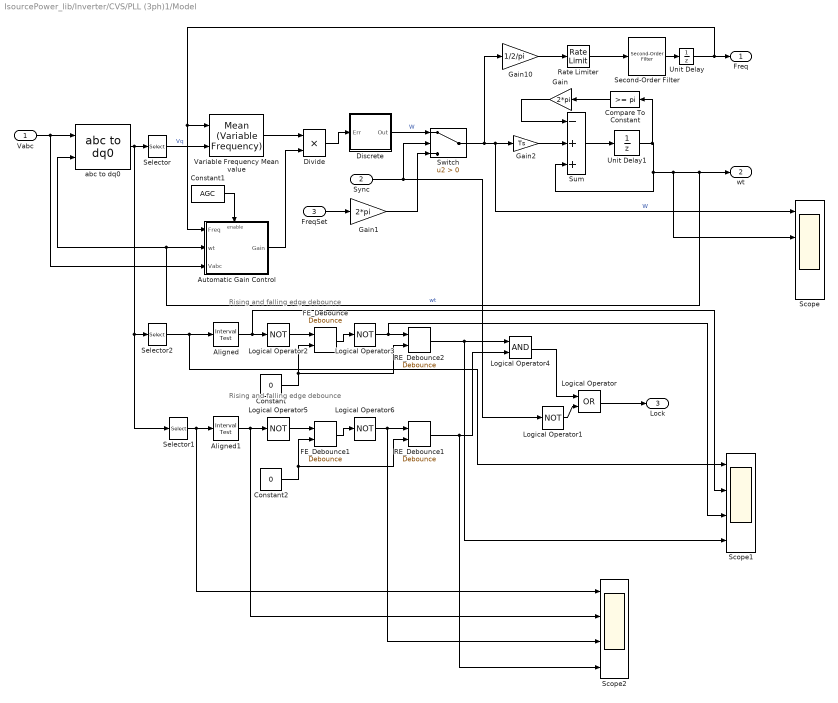
== system IsourcePower_lib/Inverter/CVS/PLL (3ph)1/Model ==
  note: Rising and falling edge debounce
  note: Rising and falling edge debounce
  Vabc : Inport  PortDimensions=3
  Sync : Inport  Port=2
  FreqSet : Inport  Port=3
  Aligned : simulink/Logic and Bit Operations/Interval Test  IntervalClosedRight=on  uplimit=0.05  IntervalClosedLeft=on  lowlimit=-0.05  OutDataTypeStr=boolean
  Aligned1 : simulink/Logic and Bit Operations/Interval Test  IntervalClosedRight=on  uplimit=1.15  IntervalClosedLeft=on  lowlimit=0.85  OutDataTypeStr=boolean
  Automatic Gain Control : Subsystem  TreatAsAtomicUnit=on
  Compare To Constant : simulink/Logic and Bit Operations/Compare To Constant  relop=>=  const=pi  OutDataTypeStr=uint8
  Constant : Constant  Value=0
  Constant1 : Constant  Value=AGC  SampleTime=Ts
  Constant2 : Constant  Value=0
  Discrete : Subsystem  DialogController=POWERSYS.PowerSysDialog  VariantControl=PID_Discrete  mask(Discrete PID Controller){Kp=ParK(1), Ki=ParK(2), Kd=ParK(3), TcD=TcD, Par_Limits=[inf 0], Init=2*pi*Par_Init(2), Ts=Ts}
      mask prompts: Kp "Proportional gain (Kp):"; Ki "Integral gain (Ki):"; Kd "Derivative gain (Kd):"; TcD "Time constant for derivative filter (s):"; Par_Limits "Output limits: [ Upper   Lower ]"; Init "Output initial value:"; Ts "Sample time:"
      mask help: This block implements a discrete PID controller.
      mask Display: disp('PID');
  Divide : Product
  FE_Debounce : debounce_lib/Debounce  Ts=sampdT  Td=paramPLLQFEDebounceTime
  FE_Debounce1 : debounce_lib/Debounce  Ts=sampdT  Td=paramPLLQFEDebounceTime
  Gain : Gain  Gain=2*pi  OutDataTypeStr=double
  Gain1 : Gain  Gain=2*pi  SaturateOnIntegerOverflow=on  OutDataTypeStr=Inherit: Same as input  ParamDataTypeStr=Inherit: Same as input
  Gain10 : Gain  Gain=1/2/pi  SaturateOnIntegerOverflow=on  OutDataTypeStr=Inherit: Same as input  ParamDataTypeStr=Inherit: Same as input
  Gain2 : Gain  Gain=Ts  SaturateOnIntegerOverflow=on  OutDataTypeStr=Inherit: Same as input  ParamDataTypeStr=Inherit: Same as input
  Logical Operator : Logic  Operator=OR  AllPortsSameDT=off  OutDataTypeStr=boolean
  Logical Operator1 : Logic  Operator=NOT  AllPortsSameDT=off  OutDataTypeStr=boolean
  Logical Operator{2..3,5..6} (4 alike) : Logic  Operator=NOT  Inputs=1  AllPortsSameDT=off  OutDataTypeStr=boolean
  Logical Operator4 : Logic  AllPortsSameDT=off  OutDataTypeStr=boolean
  RE_Debounce1 : debounce_lib/Debounce  Ts=sampdT  Td=paramPLLQREDebounceTime
  RE_Debounce2 : debounce_lib/Debounce  Ts=sampdT  Td=paramPLLQREDebounceTime
  Rate Limiter : RateLimiter  RisingSlewLimit=MaxRateChangeFreq  FallingSlewLimit=-MaxRateChangeFreq  SampleTimeMode=inherited  InitialCondition=Par_Init(2)
  Scope : Scope  NumInputPorts=4
      settings: YMin=-5~-5~-5~-5  YMax=5~5~5~5  SaveName=ScopeData4
  Scope1 : Scope  NumInputPorts=4
      settings: YMin=-0.01~0.95~0.95~-5  YMax=0.0125~1.05~1.05~5  SaveName=ScopeData5
  Scope2 : Scope  NumInputPorts=4
      settings: YMin=-5~-5~-5~-5  YMax=5~5~5~5  SaveName=ScopeData8
  Second-Order Filter : powerlib_meascontrol/Filters/Second-Order Filter  FilterType=Lowpass  Fo=FilterCutOffFreq  Zeta=0.707  Ts=Ts  Initialize=on  Vac_Init=[0 0 Par_Init(2)]  Vdc_Init=Par_Init(2)  PlotResponse=off  FreqRange=[1 500 1]
  Selector : Selector  InputPortWidth=3  IndexOptions=Index vector (dialog)  Indices=2  OutputSizes=1
  Selector1 : Selector  InputPortWidth=3  IndexOptions=Index vector (dialog)  Indices=1  OutputSizes=1
  Selector2 : Selector  InputPortWidth=3  IndexOptions=Index vector (dialog)  Indices=2  OutputSizes=1
  Sum : Sum  Inputs=-++
  Switch : Switch  Criteria=u2 > Threshold
  Unit Delay : UnitDelay  InitialCondition=Par_Init(2)  SampleTime=Ts
  Unit Delay1 : UnitDelay  SampleTime=-1
  Variable Frequency Mean value : powerlib_meascontrol/Measurements/Mean (Variable Frequency)  Finit=Par_Init(2)  Fmin=Fmin  Vinit=0  Ts=Ts
  abc to dq0 : powerlib_meascontrol/Transformations/abc to dq0  Alignment=90 degrees behind phase A axis
  Freq : Outport
  wt : Outport  Port=2
  Lock : Outport  Port=3
  wires:
  Selector2/1 -> Aligned/1, Scope1/1
  Gain/1 -> Sum/1
  Compare To Constant/1 -> Gain/1
  Unit Delay1/1 -> Sum/3, abc to dq0/2, Automatic Gain Control/2(wt), wt/1, Scope/2, Compare To Constant/1  "wt"
  Gain2/1 -> Sum/2
  Sum/1 -> Unit Delay1/1
  Logical Operator4/1 -> Logical Operator/1
  RE_Debounce1/1 -> Logical Operator4/2, Scope2/4
  Selector1/1 -> Aligned1/1, Scope2/1
  Aligned1/1 -> Logical Operator5/1, Scope2/2
  Constant2/1 -> RE_Debounce1/2, FE_Debounce1/2
  Logical Operator6/1 -> RE_Debounce1/1, Scope2/3
  FE_Debounce1/1 -> Logical Operator6/1
  Logical Operator5/1 -> FE_Debounce1/1
  RE_Debounce2/1 -> Logical Operator4/1, Scope1/4
  Aligned/1 -> Logical Operator2/1, Scope1/2
  Constant/1 -> FE_Debounce/2, RE_Debounce2/2
  Logical Operator3/1 -> RE_Debounce2/1, Scope1/3
  FE_Debounce/1 -> Logical Operator3/1
  Logical Operator2/1 -> FE_Debounce/1
  Logical Operator1/1 -> Logical Operator/2
  Logical Operator/1 -> Lock/1
  Gain1/1 -> Switch/3
  Discrete/1(Out) -> Switch/1  "W"
  Sync/1 -> Switch/2, Logical Operator1/1
  FreqSet/1 -> Gain1/1
  Unit Delay/1 -> Freq/1, Automatic Gain Control/1(Freq), Variable Frequency Mean value/1
  Rate Limiter/1 -> Second-Order Filter/1
  Gain10/1 -> Rate Limiter/1
  Selector/1 -> Variable Frequency Mean value/2  "Vq"
  Second-Order Filter/1 -> Unit Delay/1
  abc to dq0/1 -> Selector/1, Selector1/1, Selector2/1
  Vabc/1 -> abc to dq0/1, Automatic Gain Control/3(Vabc)
  Switch/1 -> Gain2/1, Scope/1, Gain10/1  "W"
  Variable Frequency Mean value/1 -> Divide/1
  Automatic Gain Control/1(Gain) -> Divide/2
  Divide/1 -> Discrete/1(Err)
  Constant1/1 -> Automatic Gain Control/Enable

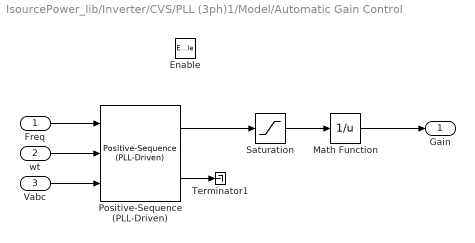
== system IsourcePower_lib/Inverter/CVS/PLL (3ph)1/Model/Automatic Gain Control ==
  Freq : Inport
  wt : Inport  Port=2
  Vabc : Inport  Port=3
  Enable : EnablePort  PropagateVarSize=During execution
  Math Function : Math  Operator=reciprocal  SaturateOnIntegerOverflow=on
  Positive-Sequence (PLL-Driven) : powerlib_meascontrol/Measurements/Positive-Sequence (PLL-Driven)  Finit=Par_Init(2)  Fmin=Fmin  InInit=[1 0]  Ts=Ts
  Saturation : Saturate  UpperLimit=inf  LowerLimit=eps
  Terminator1 : Terminator
  Gain : Outport  InitialOutput=[1]
  wires:
  Positive-Sequence (PLL-Driven)/1 -> Saturation/1
  Positive-Sequence (PLL-Driven)/2 -> Terminator1/1
  wt/1 -> Positive-Sequence (PLL-Driven)/2
  Math Function/1 -> Gain/1
  Vabc/1 -> Positive-Sequence (PLL-Driven)/3
  Freq/1 -> Positive-Sequence (PLL-Driven)/1
  Saturation/1 -> Math Function/1

== system IsourcePower_lib/Inverter/CVS/PLL (3ph)1/Model/Discrete ==
  Err : Inport  SampleTime=Ts
  "Discrete Derivative " : DiscreteTransferFcn  Numerator="[ 1  -1 ]*Kd"  Denominator="[ TcD  Ts-TcD ]"  SampleTime=Ts
  Discrete-Time Integrator : DiscreteIntegrator  gainval=Ki  InitialCondition=Init  SampleTime=Ts  LimitOutput=on  UpperSaturationLimit=Par_Limits(1)  LowerSaturationLimit=Par_Limits(2)  ICPrevOutput=DiscIntNeverNeededParam  ICPrevScaledInput=DiscIntNeverNeededParam
  Kp4 : Gain  Gain=Kp  SampleTime=Ts  SaturateOnIntegerOverflow=on  OutDataTypeStr=Inherit: Same as input  ParamDataTypeStr=Inherit: Same as input
  Saturation1 : Saturate  UpperLimit=Par_Limits(1)  LowerLimit=Par_Limits(2)  SampleTime=Ts
  Sum6 : Sum  Inputs=+++  SampleTime=Ts  SaturateOnIntegerOverflow=on  InputSameDT=on  OutDataTypeStr=Inherit: Same as first input
  Out : Outport  SampleTime=Ts  InitialOutput=0
  wires:
  "Discrete Derivative "/1 -> Sum6/3
  Discrete-Time Integrator/1 -> Sum6/2
  Kp4/1 -> Sum6/1
  Sum6/1 -> Saturation1/1
  Err/1 -> Kp4/1, Discrete-Time Integrator/1, "Discrete Derivative "/1
  Saturation1/1 -> Out/1
